simulink model "exp3_q34"  (R2019a)
settings: Solver=FixedStepAuto  StartTime=0.0  StopTime=1e-1  FixedStep=1e-7  RelTol=1e-3
libraries: dsparch4 x2
settings Model: Creator=marco  LastModifiedBy=marco
settings DebuggingCC: SigSpecEnsureSampleTimeMsg=none

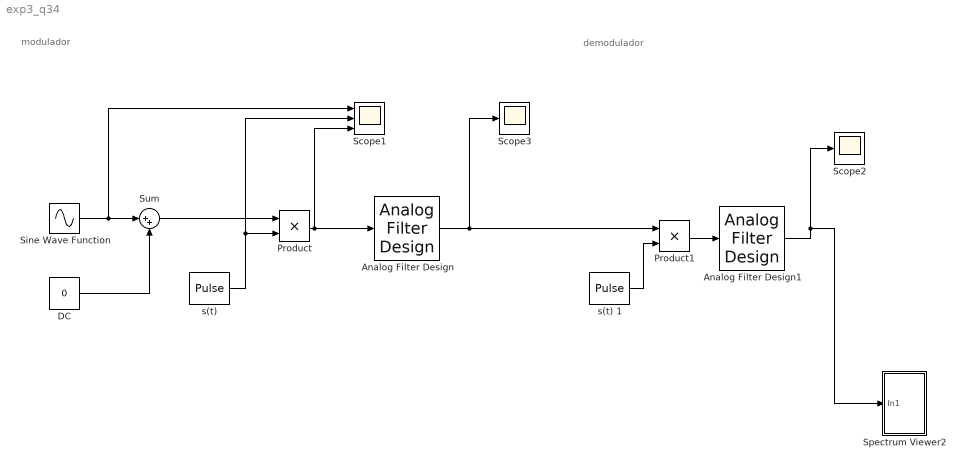
== system exp3_q34 ==
  note: demodulador
  note: modulador
  Analog Filter Design : dsparch4/Analog Filter Design  method=Butterworth  filttype=Bandpass  N=10  Wlo=2*pi*980e3  Whi=2*pi*1020e3  Rp=2  Rs=40
  Analog Filter Design1 : dsparch4/Analog Filter Design  method=Butterworth  filttype=Lowpass  N=10  Wlo=2*pi*500e3  Whi=2*pi*1020e3  Rp=2  Rs=40
  DC : Constant  Value=0
  Product : Product
  Product1 : Product
  Scope1 : Scope  NumInputPorts=3
  Scope2 : Scope
  Scope3 : Scope
  Sine Wave Function : Sin  Amplitude=0.5  Frequency=2*pi*10e3  SampleTime=0
  Spectrum Viewer2 : Subsystem
  Sum : Sum  Inputs=|++
  "s(t) " : DiscretePulseGenerator  PulseType=Time based  Period=1e-6  PulseWidth=50
  s(t) 1 : DiscretePulseGenerator  PulseType=Time based  Period=1e-6  PulseWidth=50  PhaseDelay=5e-5
  wires:
  Product/1 -> Scope1/3, Analog Filter Design/1
  Sum/1 -> Product/1
  Sine Wave Function/1 -> Scope1/1, Sum/1
  DC/1 -> Sum/2
  "s(t) "/1 -> Scope1/2, Product/2
  Analog Filter Design1/1 -> Spectrum Viewer2/1(In1), Scope2/1
  Analog Filter Design/1 -> Product1/1, Scope3/1
  Product1/1 -> Analog Filter Design1/1
  s(t) 1/1 -> Product1/2

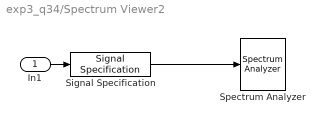
== system exp3_q34/Spectrum Viewer2 ==
  In1 : Inport
  Signal Specification : SignalSpecification  SampleTime=1e-5
  Spectrum Analyzer : SpectrumAnalyzer
  wires:
  In1/1 -> Signal Specification/1
  Signal Specification/1 -> Spectrum Analyzer/1
